simulink model "r5"  (Simulink 8.6)
settings: Solver=FixedStepAuto  StartTime=0.0  StopTime=10.0  RelTol=1e-3
undefined symbols (not defined in the file): dt, sldvsubsys, transition_v, transition_y
libraries: simulink x2, sldvlib x2
settings Model: Creator=elliocm  LastModifiedBy=mike
settings DebuggingCC: FcnCallInpInsideContextMsg=UseLocalSettings

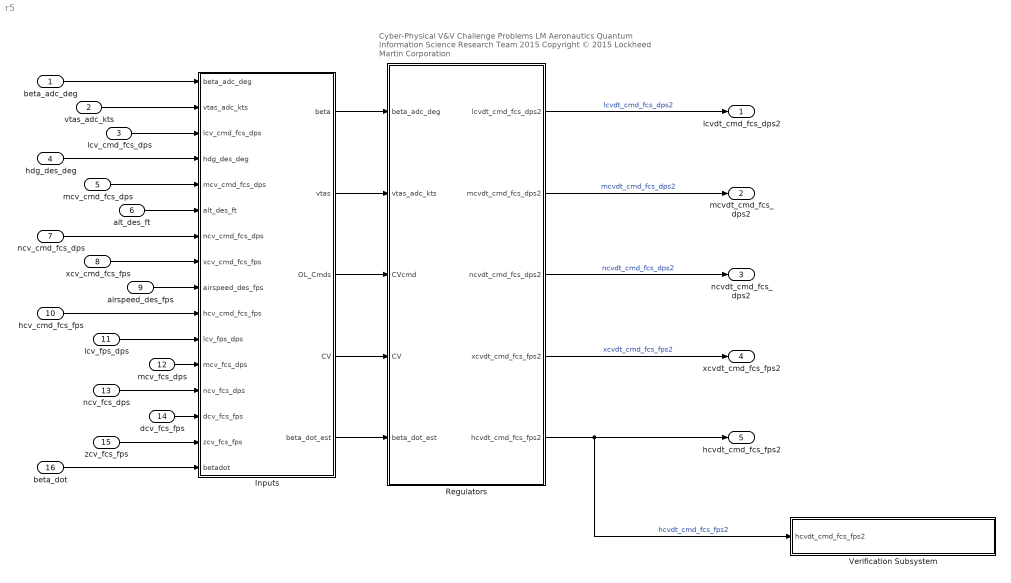
== system r5 ==
  note: Cyber-Physical V&V Challenge Problems
      | LM Aeronautics Quantum Information Science Research Team 2015
      | Copyright © 2015 Lockheed Martin Corporation
  beta_adc_deg : Inport  OutDataTypeStr=double
  vtas_adc_kts : Inport  Port=2  OutDataTypeStr=double
  "lcv_cmd_fcs_dps " : Inport  Port=3  OutDataTypeStr=double
  hdg_des_deg : Inport  Port=4  OutDataTypeStr=double
  mcv_cmd_fcs_dps : Inport  Port=5  OutDataTypeStr=double
  alt_des_ft : Inport  Port=6  OutDataTypeStr=double
  ncv_cmd_fcs_dps : Inport  Port=7  OutDataTypeStr=double
  xcv_cmd_fcs_fps : Inport  Port=8  OutDataTypeStr=double
  airspeed_des_fps : Inport  Port=9  OutDataTypeStr=double
  hcv_cmd_fcs_fps : Inport  Port=10  OutDataTypeStr=double
  lcv_fps_dps : Inport  Port=11  OutDataTypeStr=double
  mcv_fcs_dps : Inport  Port=12  OutDataTypeStr=double
  ncv_fcs_dps : Inport  Port=13  OutDataTypeStr=double
  dcv_fcs_fps : Inport  Port=14  OutDataTypeStr=double
  zcv_fcs_fps : Inport  Port=15  OutDataTypeStr=double
  beta_dot : Inport  Port=16  OutDataTypeStr=double
  Inputs : Subsystem
  Regulators : Subsystem
  Verification Subsystem : Subsystem  Tag=VerificationSubsystem  DisableCoverage=on  LoadFcn=sldvsubsys('check')  TreatAsAtomicUnit=on  SimViewingDevice=on  mask(VerificationSubsystem){}
      mask init:
      | sldvsubsys('maskInit');
      settings: CopyFcn=sldvsubsys('copy');  OpenFcn=open_system(gcb,'force');
      settings: PreSaveFcn=|
      | set_param(gcb,'SimViewingDevice','on');
      | sldvsubsys('check');
      mask Help: helpview(fullfile(docroot,'toolbox','sldv','sldv.map'),'verificationsubsystem')
      mask Display: image(imread('sldvicon_versubsys.png','BackGroundColor',[1 1 1]),'center');
  lcvdt_cmd_fcs_dps2 : Outport
  mcvdt_cmd_fcs_dps2 : Outport  Port=2
  ncvdt_cmd_fcs_dps2 : Outport  Port=3
  xcvdt_cmd_fcs_fps2 : Outport  Port=4
  hcvdt_cmd_fcs_fps2 : Outport  Port=5
  wires:
  Inputs/4(CV) -> Regulators/4(CV)
  Inputs/3(OL_Cmds) -> Regulators/3(CVcmd)
  Inputs/1(beta) -> Regulators/1(beta_adc_deg)
  Inputs/5(beta_dot_est) -> Regulators/5(beta_dot_est)
  beta_adc_deg/1 -> Inputs/1(beta_adc_deg)
  vtas_adc_kts/1 -> Inputs/2(vtas_adc_kts)
  "lcv_cmd_fcs_dps "/1 -> Inputs/3("lcv_cmd_fcs_dps ")
  mcv_cmd_fcs_dps/1 -> Inputs/5(mcv_cmd_fcs_dps)
  ncv_cmd_fcs_dps/1 -> Inputs/7(ncv_cmd_fcs_dps)
  xcv_cmd_fcs_fps/1 -> Inputs/8(xcv_cmd_fcs_fps)
  hcv_cmd_fcs_fps/1 -> Inputs/10(hcv_cmd_fcs_fps)
  hdg_des_deg/1 -> Inputs/4(hdg_des_deg)
  alt_des_ft/1 -> Inputs/6(alt_des_ft)
  airspeed_des_fps/1 -> Inputs/9(airspeed_des_fps)
  Regulators/1(lcvdt_cmd_fcs_dps2) -> lcvdt_cmd_fcs_dps2/1  "lcvdt_cmd_fcs_dps2"
  Regulators/2(mcvdt_cmd_fcs_dps2) -> mcvdt_cmd_fcs_dps2/1  "mcvdt_cmd_fcs_dps2"
  Regulators/3(ncvdt_cmd_fcs_dps2) -> ncvdt_cmd_fcs_dps2/1  "ncvdt_cmd_fcs_dps2"
  Regulators/5(hcvdt_cmd_fcs_fps2) -> Verification Subsystem/1(hcvdt_cmd_fcs_fps2), hcvdt_cmd_fcs_fps2/1  "hcvdt_cmd_fcs_fps2"
  Regulators/4(xcvdt_cmd_fcs_fps2) -> xcvdt_cmd_fcs_fps2/1  "xcvdt_cmd_fcs_fps2"
  zcv_fcs_fps/1 -> Inputs/15(zcv_fcs_fps)
  dcv_fcs_fps/1 -> Inputs/14(dcv_fcs_fps)
  lcv_fps_dps/1 -> Inputs/11(lcv_fps_dps)
  mcv_fcs_dps/1 -> Inputs/12(mcv_fcs_dps)
  ncv_fcs_dps/1 -> Inputs/13(ncv_fcs_dps)
  beta_dot/1 -> Inputs/16(betadot)
  Inputs/2(vtas) -> Regulators/2(vtas_adc_kts)

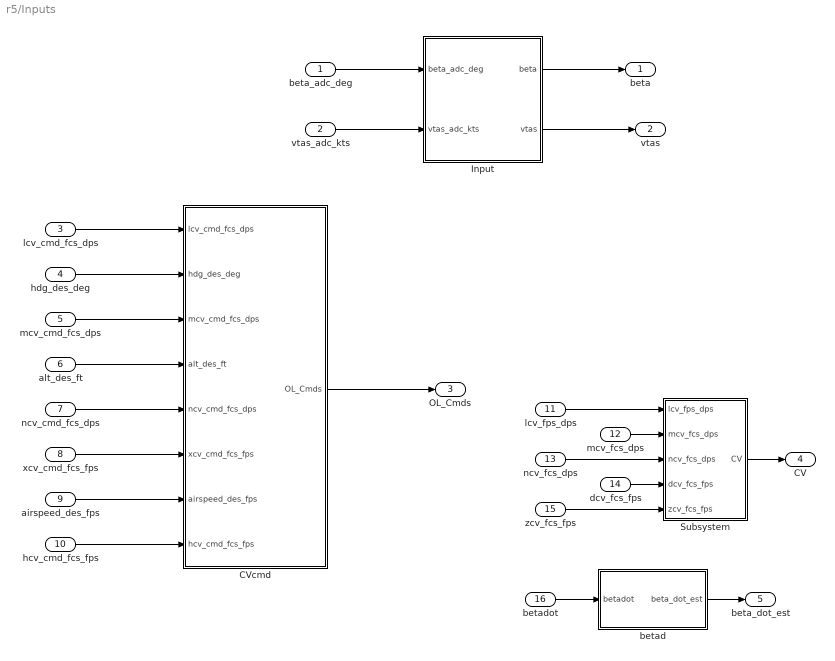
== system r5/Inputs ==
  beta_adc_deg : Inport
  vtas_adc_kts : Inport  Port=2
  "lcv_cmd_fcs_dps " : Inport  Port=3
  hdg_des_deg : Inport  Port=4
  mcv_cmd_fcs_dps : Inport  Port=5
  alt_des_ft : Inport  Port=6
  ncv_cmd_fcs_dps : Inport  Port=7
  xcv_cmd_fcs_fps : Inport  Port=8
  airspeed_des_fps : Inport  Port=9
  hcv_cmd_fcs_fps : Inport  Port=10
  lcv_fps_dps : Inport  Port=11
  mcv_fcs_dps : Inport  Port=12
  ncv_fcs_dps : Inport  Port=13
  dcv_fcs_fps : Inport  Port=14
  zcv_fcs_fps : Inport  Port=15
  betadot : Inport  Port=16
  CVcmd : Subsystem
  Input : Subsystem
  Subsystem : Subsystem
  betad : Subsystem
  beta : Outport
  vtas : Outport  Port=2
  OL_Cmds : Outport  Port=3
  CV : Outport  Port=4
  beta_dot_est : Outport  Port=5
  wires:
  Subsystem/1(CV) -> CV/1
  CVcmd/1(OL_Cmds) -> OL_Cmds/1
  beta_adc_deg/1 -> Input/1(beta_adc_deg)
  vtas_adc_kts/1 -> Input/2(vtas_adc_kts)
  "lcv_cmd_fcs_dps "/1 -> CVcmd/1("lcv_cmd_fcs_dps ")
  mcv_cmd_fcs_dps/1 -> CVcmd/3(mcv_cmd_fcs_dps)
  ncv_cmd_fcs_dps/1 -> CVcmd/5(ncv_cmd_fcs_dps)
  xcv_cmd_fcs_fps/1 -> CVcmd/6(xcv_cmd_fcs_fps)
  hcv_cmd_fcs_fps/1 -> CVcmd/8(hcv_cmd_fcs_fps)
  hdg_des_deg/1 -> CVcmd/2(hdg_des_deg)
  alt_des_ft/1 -> CVcmd/4(alt_des_ft)
  airspeed_des_fps/1 -> CVcmd/7(airspeed_des_fps)
  zcv_fcs_fps/1 -> Subsystem/5(zcv_fcs_fps)
  dcv_fcs_fps/1 -> Subsystem/4(dcv_fcs_fps)
  lcv_fps_dps/1 -> Subsystem/1(lcv_fps_dps)
  mcv_fcs_dps/1 -> Subsystem/2(mcv_fcs_dps)
  ncv_fcs_dps/1 -> Subsystem/3(ncv_fcs_dps)
  betadot/1 -> betad/1(betadot)
  betad/1(beta_dot_est) -> beta_dot_est/1
  Input/1(beta) -> beta/1
  Input/2(vtas) -> vtas/1

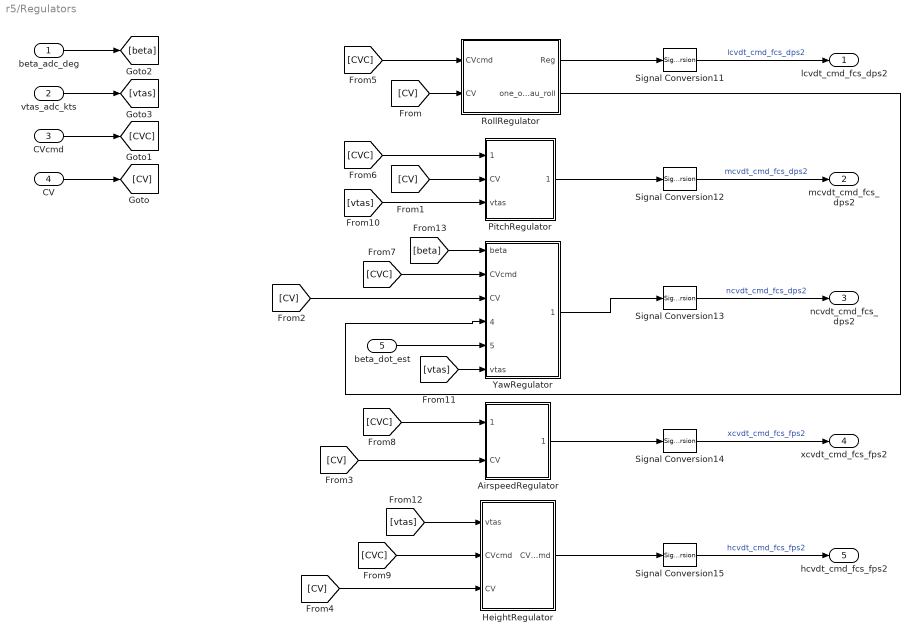
== system r5/Regulators ==
  beta_adc_deg : Inport
  vtas_adc_kts : Inport  Port=2
  CVcmd : Inport  Port=3
  CV : Inport  Port=4
  beta_dot_est : Inport  Port=5
  AirspeedRegulator : Subsystem
  HeightRegulator : Subsystem
  PitchRegulator : Subsystem
  RollRegulator : Subsystem
  Signal Conversion{11..15} (5 alike) : SignalConversion  ConversionOutput=Contiguous copy  OverrideOpt=on
  YawRegulator : Subsystem
  lcvdt_cmd_fcs_dps2 : Outport
  mcvdt_cmd_fcs_dps2 : Outport  Port=2
  ncvdt_cmd_fcs_dps2 : Outport  Port=3
  xcvdt_cmd_fcs_fps2 : Outport  Port=4
  hcvdt_cmd_fcs_fps2 : Outport  Port=5
  wires:
  RollRegulator/1(Reg) -> Signal Conversion11/1
  PitchRegulator/1(CVdt_cmd) -> Signal Conversion12/1
  YawRegulator/1(CVdt_cmd) -> Signal Conversion13/1
  AirspeedRegulator/1(CVdt_cmd) -> Signal Conversion14/1
  HeightRegulator/1(CVdt_cmd) -> Signal Conversion15/1
  [CVC] -> HeightRegulator/2(CVcmd)
  [CVC] -> YawRegulator/2(CVcmd)
  Signal Conversion11/1 -> lcvdt_cmd_fcs_dps2/1  "lcvdt_cmd_fcs_dps2"
  Signal Conversion12/1 -> mcvdt_cmd_fcs_dps2/1  "mcvdt_cmd_fcs_dps2"
  Signal Conversion13/1 -> ncvdt_cmd_fcs_dps2/1  "ncvdt_cmd_fcs_dps2"
  Signal Conversion15/1 -> hcvdt_cmd_fcs_fps2/1  "hcvdt_cmd_fcs_fps2"
  Signal Conversion14/1 -> xcvdt_cmd_fcs_fps2/1  "xcvdt_cmd_fcs_fps2"
  RollRegulator/2(one_over_Tau_roll) -> YawRegulator/4(one_over_Tau_roll)
  beta_dot_est/1 -> YawRegulator/5(beta_dot_est)
  CV/1 -> [CV]
  [CV] -> RollRegulator/2(CV)
  [CV] -> PitchRegulator/2(CV)
  [CV] -> YawRegulator/3(CV)
  [CV] -> AirspeedRegulator/2(CV)
  [CV] -> HeightRegulator/3(CV)
  CVcmd/1 -> [CVC]
  [CVC] -> RollRegulator/1(CVcmd)
  [CVC] -> PitchRegulator/1(CV_cmd)
  [CVC] -> AirspeedRegulator/1(CVcmd)
  [vtas] -> PitchRegulator/3(vtas)
  [vtas] -> HeightRegulator/1(vtas)
  beta_adc_deg/1 -> [beta]
  vtas_adc_kts/1 -> [vtas]
  [vtas] -> YawRegulator/6(vtas)
  [beta] -> YawRegulator/1(beta)

== system r5/Verification Subsystem ==
  note: The Inner Loop Height Regulator Shall not command translational height accelerations greater
      | than the capability of the system (32 ft/sec2) for durations exceeding 100 frames (1 second @ 100 hz).
  note: hcvdt_cmd_fcs_fps2{t}<=32 or hcvdt_cmd_fcs_fps2{t-1}<=32 or hcvdt_cmd_fcs_fps2{t-2}<=32 or hcvdt_cmd_fcs_fps2{t-3}<=32 or hcvdt_cmd_fcs_fps2{t-4}<=32 or hcvdt_cmd_fcs_fps2{t-5}<=32 or hcvdt_cmd_fcs_fps2{t-6}<=32 or hcvdt_cmd_fcs_fps2{t-7}<=32 or hcvdt_cmd_fcs_fps2{t-8}<=32 or hcvdt_cmd_fcs_fps2{t-9}<=32 or hcvdt_cmd_fcs_fps2{t-10}<=32 or hcvdt_cmd_fcs_fps2{t-11}<=32 or hcvdt_cmd_fcs_fps2{t-12}<=32 or hcvdt_cmd_fcs_fps2{t-13}<=32 or hcvdt_cmd_fcs_fps2{t-14}<=32 or hcvdt_cmd_fcs_fps2{t-15}<=32 or hcvdt_cmd_fcs_fps2{t-16}<=32 or hcvdt_cmd_fcs_fps2{t-17}<=32 or hcvdt_cmd_fcs_fps2{t-18}<=32 or hcvdt_cmd_fcs_fps2{t-19}<=32 or hcvdt_cmd_fcs_fps2{t-20}<=32 or hcvdt_cmd_fcs_fps2{t-21}<=32 or hcvdt_cmd_fcs_fps2{t-22}<=32 or hcvdt_cmd_fcs_fps2{t-23}<=32 or hcvdt_cmd_fcs_fps2{t-24}<=32 or hcvdt_cmd_fcs_fps2{t-25}<=32 or hcvdt_cmd_fcs_fps2{t-26}<=32 or hcvdt_cmd_fcs_fps2{t-27}<=32 or hcvdt_cmd_fcs_fps2{t-28}<=32 or hcvdt_cmd_fcs_fps2{t-29}<=32 or hcvdt_cmd_fcs_fps2{t-30}<=32 or hcvdt_cmd_fcs_fps2{t-31}<=32 or hcvdt_cmd_fcs_fps2{t-32}<=32 or hcvdt_cmd_fcs_fps2{t-33}<=32 or hcvdt_cmd_fcs_fps2{t-34}<=32 or hcvdt_cmd_fcs_fps2{t-35}<=32 or hcvdt_cmd_fcs_fps2{t-36}<=32 or hcvdt_cmd_fcs_fps2{t-37}<=32 or hcvdt_cmd_fcs_fps2{t-38}<=32 or hcvdt_cmd_fcs_fps2{t-39}<=32 or hcvdt_cmd_fcs_fps2{t-40}<=32 or hcvdt_cmd_fcs_fps2{t-41}<=32 or hcvdt_cmd_fcs_fps2{t-42}<=32 or hcvdt_cmd_fcs_fps2{t-43}<=32 or hcvdt_cmd_fcs_fps2{t-44}<=32 or hcvdt_cmd_fcs_fps2{t-45}<=32 or hcvdt_cmd_fcs_fps2{t-46}<=32 or hcvdt_cmd_fcs_fps2{t-47}<=32 or hcvdt_cmd_fcs_fps2{t-48}<=32 or hcvdt_cmd_fcs_fps2{t-49}<=32 or hcvdt_cmd_fcs_fps2{t-32}<=32 or hcvdt_cmd_fcs_fps2{t-51}<=32 or hcvdt_cmd_fcs_fps2{t-52}<=32 or hcvdt_cmd_fcs_fps2{t-53}<=32 or hcvdt_cmd_fcs_fps2{t-54}<=32 or hcvdt_cmd_fcs_fps2{t-55}<=32 or hcvdt_cmd_fcs_fps2{t-56}<=32 or hcvdt_cmd_fcs_fps2{t-57}<=32 or hcvdt_cmd_fcs_fps2{t-58}<=32 or hcvdt_cmd_fcs_fps2{t-59}<=32 or hcvdt_cmd_fcs_fps2{t-60}<=32 or hcvdt_cmd_fcs_fps2{t-61}<=32 or hcvdt_cmd_fcs_fps2{t-62}<=32 or hcvdt_cmd_fcs_fps2{t-63}<=32 or hcvdt_cmd_fcs_fps2{t-64}<=32 or hcvdt_cmd_fcs_fps2{t-65}<=32 or hcvdt_cmd_fcs_fps2{t-66}<=32 or hcvdt_cmd_fcs_fps2{t-67}<=32 or hcvdt_cmd_fcs_fps2{t-68}<=32 or hcvdt_cmd_fcs_fps2{t-69}<=32 or hcvdt_cmd_fcs_fps2{t-70}<=32 or hcvdt_cmd_fcs_fps2{t-71}<=32 or hcvdt_cmd_fcs_fps2{t-72}<=32 or hcvdt_cmd_fcs_fps2{t-73}<=32 or hcvdt_cmd_fcs_fps2{t-74}<=32 or hcvdt_cmd_fcs_fps2{t-75}<=32 or hcvdt_cmd_fcs_fps2{t-76}<=32 or hcvdt_cmd_fcs_fps2{t-77}<=32 or hcvdt_cmd_fcs_fps2{t-78}<=32 or hcvdt_cmd_fcs_fps2{t-79}<=32 or hcvdt_cmd_fcs_fps2{t-80}<=32 or hcvdt_cmd_fcs_fps2{t-81}<=32 or hcvdt_cmd_fcs_fps2{t-82}<=32 or hcvdt_cmd_fcs_fps2{t-83}<=32 or hcvdt_cmd_fcs_fps2{t-84}<=32 or hcvdt_cmd_fcs_fps2{t-85}<=32 or hcvdt_cmd_fcs_fps2{t-86}<=32 or hcvdt_cmd_fcs_fps2{t-87}<=32 or hcvdt_cmd_fcs_fps2{t-88}<=32 or hcvdt_cmd_fcs_fps2{t-89}<=32 or hcvdt_cmd_fcs_fps2{t-90}<=32 or hcvdt_cmd_fcs_fps2{t-91}<=32 or hcvdt_cmd_fcs_fps2{t-92}<=32 or hcvdt_cmd_fcs_fps2{t-93}<=32 or hcvdt_cmd_fcs_fps2{t-94}<=32 or hcvdt_cmd_fcs_fps2{t-95}<=32 or hcvdt_cmd_fcs_fps2{t-96}<=32 or hcvdt_cmd_fcs_fps2{t-97}<=32 or hcvdt_cmd_fcs_fps2{t-98}<=32 or hcvdt_cmd_fcs_fps2{t-99}<=32;
  hcvdt_cmd_fcs_fps2 : Inport
  Constant : Constant  Value=32
  Detector : sldvlib/Temporal Operators/Detector  reset=off  typ=Synchronized  in_hold=100  delay=1  out_hold=3
  Logical Operator : Logic  Operator=NOT  AllPortsSameDT=off  OutDataTypeStr=boolean
  Proof Objective : sldvlib/Objectives and Constraints/Proof Objective  enabled=on  customAVTBlockType=Proof Objective  intervals=true  dispValues=on  outEnabled=off  enableStopSim=off
      settings: AttributesFormatString=%<intervals>
  Relational Operator : RelationalOperator  Operator=>  OutDataTypeStr=boolean
  wires:
  Relational Operator/1 -> Detector/1
  hcvdt_cmd_fcs_fps2/1 -> Relational Operator/1
  Constant/1 -> Relational Operator/2
  Logical Operator/1 -> Proof Objective/1
  Detector/1 -> Logical Operator/1

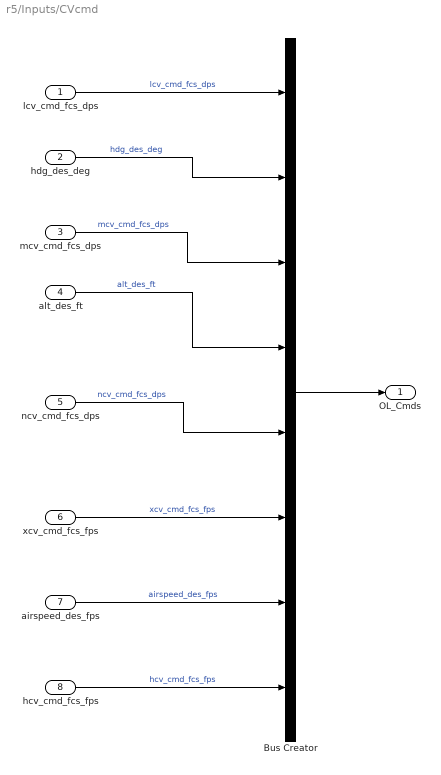
== system r5/Inputs/CVcmd ==
  "lcv_cmd_fcs_dps " : Inport
  hdg_des_deg : Inport  Port=2
  mcv_cmd_fcs_dps : Inport  Port=3
  alt_des_ft : Inport  Port=4
  ncv_cmd_fcs_dps : Inport  Port=5
  xcv_cmd_fcs_fps : Inport  Port=6
  airspeed_des_fps : Inport  Port=7
  hcv_cmd_fcs_fps : Inport  Port=8
  Bus Creator : BusCreator  Inputs=8
  OL_Cmds : Outport
  wires:
  "lcv_cmd_fcs_dps "/1 -> Bus Creator/1  "lcv_cmd_fcs_dps"
  mcv_cmd_fcs_dps/1 -> Bus Creator/3  "mcv_cmd_fcs_dps"
  ncv_cmd_fcs_dps/1 -> Bus Creator/5  "ncv_cmd_fcs_dps"
  xcv_cmd_fcs_fps/1 -> Bus Creator/6  "xcv_cmd_fcs_fps"
  hcv_cmd_fcs_fps/1 -> Bus Creator/8  "hcv_cmd_fcs_fps"
  Bus Creator/1 -> OL_Cmds/1
  hdg_des_deg/1 -> Bus Creator/2  "hdg_des_deg"
  alt_des_ft/1 -> Bus Creator/4  "alt_des_ft"
  airspeed_des_fps/1 -> Bus Creator/7  "airspeed_des_fps"

== system r5/Inputs/Input ==
  beta_adc_deg : Inport
  vtas_adc_kts : Inport  Port=2
  egi_fcs_in : Subsystem
  beta : Outport
  vtas : Outport  Port=2
  wires:
  beta_adc_deg/1 -> egi_fcs_in/1(beta_adc_deg)  "beta_adc_deg"
  vtas_adc_kts/1 -> egi_fcs_in/2(vtas_adc_kts)  "vtas_adc_kts"
  egi_fcs_in/1(beta_deg) -> beta/1
  egi_fcs_in/2(vtas_kts) -> vtas/1

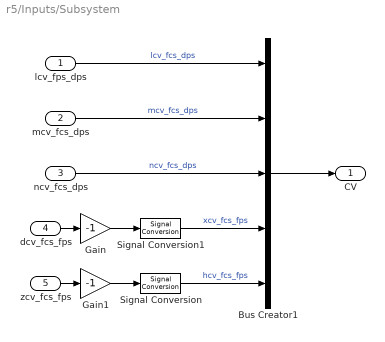
== system r5/Inputs/Subsystem ==
  lcv_fps_dps : Inport
  mcv_fcs_dps : Inport  Port=2
  ncv_fcs_dps : Inport  Port=3
  dcv_fcs_fps : Inport  Port=4
  zcv_fcs_fps : Inport  Port=5
  Bus Creator1 : BusCreator  Inputs=5
  Gain : Gain  Gain=-1
  Gain1 : Gain  Gain=-1
  Signal Conversion : SignalConversion  ConversionOutput=Contiguous copy
  Signal Conversion1 : SignalConversion  ConversionOutput=Contiguous copy
  CV : Outport
  wires:
  Gain1/1 -> Signal Conversion/1
  zcv_fcs_fps/1 -> Gain1/1
  Signal Conversion1/1 -> Bus Creator1/4  "xcv_fcs_fps"
  Gain/1 -> Signal Conversion1/1
  Bus Creator1/1 -> CV/1
  mcv_fcs_dps/1 -> Bus Creator1/2  "mcv_fcs_dps"
  lcv_fps_dps/1 -> Bus Creator1/1  "lcv_fcs_dps"
  Signal Conversion/1 -> Bus Creator1/5  "hcv_fcs_fps"
  ncv_fcs_dps/1 -> Bus Creator1/3  "ncv_fcs_dps"
  dcv_fcs_fps/1 -> Gain/1

== system r5/Inputs/betad ==
  betadot : Inport
  beta_dot_est : Outport
  wires:
  betadot/1 -> beta_dot_est/1

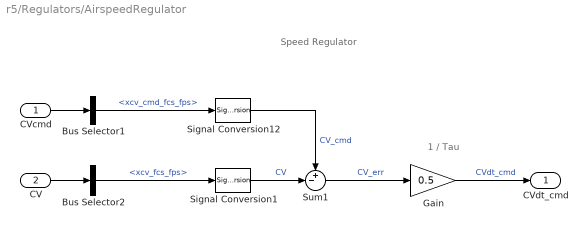
== system r5/Regulators/AirspeedRegulator ==
  note: Speed Regulator
  note: 1 / Tau
  CVcmd : Inport
  CV : Inport  Port=2
  Bus Selector1 : BusSelector  OutputSignals=xcv_cmd_fcs_fps
  Bus Selector2 : BusSelector  OutputSignals=xcv_fcs_fps
  Gain : Gain  Gain=0.5
  Signal Conversion1 : SignalConversion  ConversionOutput=Contiguous copy  OverrideOpt=on
  Signal Conversion12 : SignalConversion  ConversionOutput=Contiguous copy  OverrideOpt=on
  Sum1 : Sum  Inputs=+-|  SaturateOnIntegerOverflow=on  InputSameDT=on  OutDataTypeStr=Inherit: Same as first input
  CVdt_cmd : Outport
  wires:
  Gain/1 -> CVdt_cmd/1  "CVdt_cmd"
  CVcmd/1 -> Bus Selector1/1
  Signal Conversion12/1 -> Sum1/1  "CV_cmd"
  Signal Conversion1/1 -> Sum1/2  "CV"
  CV/1 -> Bus Selector2/1
  Bus Selector2/1 -> Signal Conversion1/1  "<xcv_fcs_fps>"
  Bus Selector1/1 -> Signal Conversion12/1  "<xcv_cmd_fcs_fps>"
  Sum1/1 -> Gain/1  "CV_err"

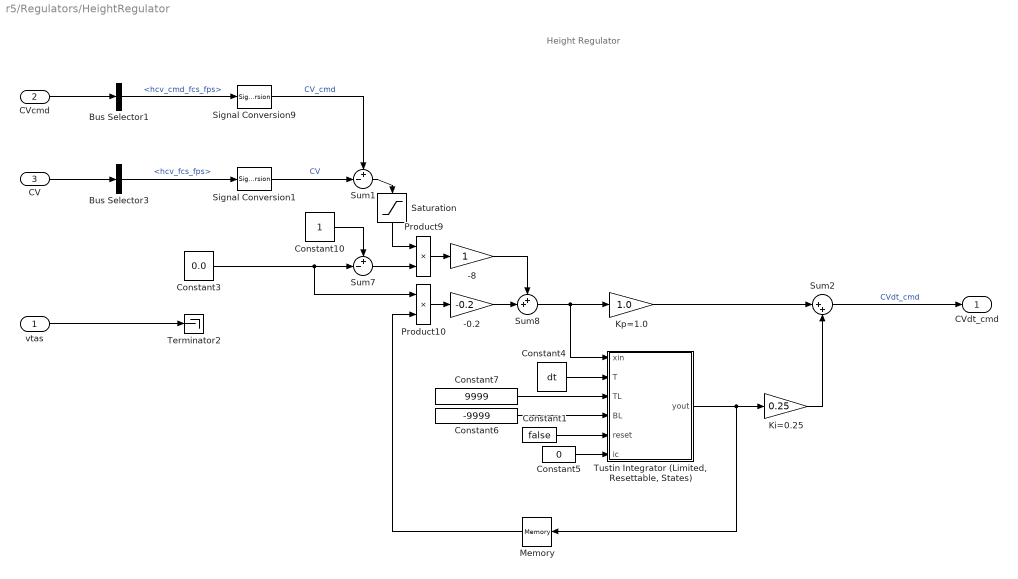
== system r5/Regulators/HeightRegulator ==
  note: Height Regulator
  vtas : Inport
  CVcmd : Inport  Port=2
  CV : Inport  Port=3
  -0.2 : Gain  Gain=-0.2
  -8 : Gain
  Bus Selector1 : BusSelector  OutputSignals=hcv_cmd_fcs_fps
  Bus Selector3 : BusSelector  OutputSignals=hcv_fcs_fps
  Constant1 : Constant  Value=false
  Constant10 : Constant
  Constant3 : Constant  Value=0.0
  Constant4 : Constant  Value=dt
  Constant5 : Constant  Value=0
  Constant6 : Constant  Value=-9999
  Constant7 : Constant  Value=9999
  Ki=0.25 : Gain  Gain=0.25
  Kp=1.0 : Gain  Gain=1.0
  Memory : Memory
  Product10 : Product  SaturateOnIntegerOverflow=on  OutDataTypeStr=Inherit: Same as first input
  Product9 : Product  SaturateOnIntegerOverflow=on  OutDataTypeStr=Inherit: Same as first input
  Saturation : Saturate  UpperLimit=1  LowerLimit=-1
  Signal Conversion1 : SignalConversion  ConversionOutput=Contiguous copy  OverrideOpt=on
  Signal Conversion9 : SignalConversion  ConversionOutput=Contiguous copy  OverrideOpt=on
  Sum1 : Sum  Inputs=+-|  SaturateOnIntegerOverflow=on  InputSameDT=on  OutDataTypeStr=Inherit: Same as first input
  Sum2 : Sum  Inputs=|++  SaturateOnIntegerOverflow=on  InputSameDT=on  OutDataTypeStr=Inherit: Same as first input
  Sum7 : Sum  Inputs=+-|
  Sum8 : Sum  Inputs=++|
  Terminator2 : Terminator
  "Tustin Integrator (Limited, Resettable, States)" : Subsystem
  CVdt_cmd : Outport
  wires:
  Bus Selector1/1 -> Signal Conversion9/1  "<hcv_cmd_fcs_fps>"
  CVcmd/1 -> Bus Selector1/1
  Signal Conversion9/1 -> Sum1/1  "CV_cmd"
  Signal Conversion1/1 -> Sum1/2  "CV"
  CV/1 -> Bus Selector3/1
  Bus Selector3/1 -> Signal Conversion1/1  "<hcv_fcs_fps>"
  Sum1/1 -> Saturation/1
  Sum2/1 -> CVdt_cmd/1  "CVdt_cmd"
  Ki=0.25/1 -> Sum2/2
  Kp=1.0/1 -> Sum2/1
  Product9/1 -> -8/1
  Product10/1 -> -0.2/1
  -0.2/1 -> Sum8/2
  -8/1 -> Sum8/1
  Sum7/1 -> Product9/2
  Constant3/1 -> Sum7/2, Product10/1
  Constant10/1 -> Sum7/1
  Sum8/1 -> "Tustin Integrator (Limited, Resettable, States)"/1(xin), Kp=1.0/1
  Memory/1 -> Product10/2
  vtas/1 -> Terminator2/1
  Saturation/1 -> Product9/1
  Constant4/1 -> "Tustin Integrator (Limited, Resettable, States)"/2(T)
  Constant7/1 -> "Tustin Integrator (Limited, Resettable, States)"/3(TL)
  Constant6/1 -> "Tustin Integrator (Limited, Resettable, States)"/4(BL)
  Constant1/1 -> "Tustin Integrator (Limited, Resettable, States)"/5(reset)
  Constant5/1 -> "Tustin Integrator (Limited, Resettable, States)"/6(ic)
  "Tustin Integrator (Limited, Resettable, States)"/1(yout) -> Memory/1, Ki=0.25/1

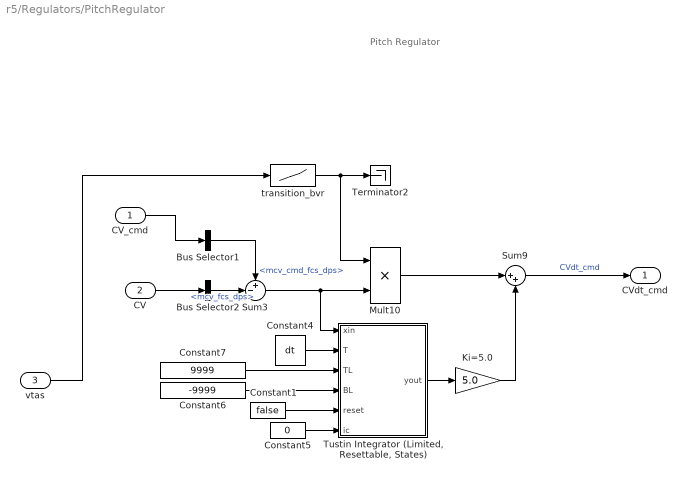
== system r5/Regulators/PitchRegulator ==
  note: Pitch Regulator
  CV_cmd : Inport
  CV : Inport  Port=2
  vtas : Inport  Port=3
  Bus Selector1 : BusSelector  OutputSignals=mcv_cmd_fcs_dps
  Bus Selector2 : BusSelector  OutputSignals=mcv_fcs_dps
  Constant1 : Constant  Value=false
  Constant4 : Constant  Value=dt
  Constant5 : Constant  Value=0
  Constant6 : Constant  Value=-9999
  Constant7 : Constant  Value=9999
  Ki=5.0 : Gain  Gain=5.0
  Mult10 : Product  SaturateOnIntegerOverflow=on  InputSameDT=on  OutDataTypeStr=Inherit: Same as first input
  Sum3 : Sum  Inputs=+-|  SaturateOnIntegerOverflow=on  InputSameDT=on  OutDataTypeStr=Inherit: Same as first input
  Sum9 : Sum  Inputs=|++  SaturateOnIntegerOverflow=on  InputSameDT=on  OutDataTypeStr=Inherit: Same as first input
  Terminator2 : Terminator
  "Tustin Integrator (Limited, Resettable, States)" : Subsystem
  transition_bvr : Lookup  InputValues=[120 185]  Table=[15 20]
  CVdt_cmd : Outport
  wires:
  CV_cmd/1 -> Bus Selector1/1
  CV/1 -> Bus Selector2/1
  Constant4/1 -> "Tustin Integrator (Limited, Resettable, States)"/2(T)
  Constant5/1 -> "Tustin Integrator (Limited, Resettable, States)"/6(ic)
  "Tustin Integrator (Limited, Resettable, States)"/1(yout) -> Ki=5.0/1
  Mult10/1 -> Sum9/1
  Ki=5.0/1 -> Sum9/2
  Sum9/1 -> CVdt_cmd/1  "CVdt_cmd"
  Bus Selector1/1 -> Sum3/1  "<mcv_cmd_fcs_dps>"
  Bus Selector2/1 -> Sum3/2  "<mcv_fcs_dps>"
  transition_bvr/1 -> Terminator2/1, Mult10/1
  Constant1/1 -> "Tustin Integrator (Limited, Resettable, States)"/5(reset)
  vtas/1 -> transition_bvr/1
  Sum3/1 -> "Tustin Integrator (Limited, Resettable, States)"/1(xin), Mult10/2
  Constant6/1 -> "Tustin Integrator (Limited, Resettable, States)"/4(BL)
  Constant7/1 -> "Tustin Integrator (Limited, Resettable, States)"/3(TL)

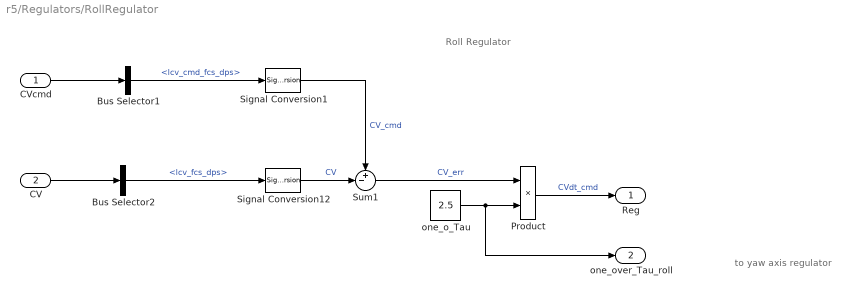
== system r5/Regulators/RollRegulator ==
  note: Roll Regulator
  note: to yaw axis regulator
  CVcmd : Inport
  CV : Inport  Port=2
  Bus Selector1 : BusSelector  OutputSignals=lcv_cmd_fcs_dps
  Bus Selector2 : BusSelector  OutputSignals=lcv_fcs_dps
  Product : Product  RndMeth=Zero
  Signal Conversion1 : SignalConversion  ConversionOutput=Contiguous copy  OverrideOpt=on
  Signal Conversion12 : SignalConversion  ConversionOutput=Contiguous copy  OverrideOpt=on
  Sum1 : Sum  Inputs=+-|  SaturateOnIntegerOverflow=on  InputSameDT=on  OutDataTypeStr=Inherit: Same as first input
  one_o_Tau : Constant  Value=2.5
  Reg : Outport
  one_over_Tau_roll : Outport  Port=2
  wires:
  Sum1/1 -> Product/1  "CV_err"
  Signal Conversion1/1 -> Sum1/1  "CV_cmd"
  Signal Conversion12/1 -> Sum1/2  "CV"
  CV/1 -> Bus Selector2/1
  Bus Selector2/1 -> Signal Conversion12/1  "<lcv_fcs_dps>"
  Bus Selector1/1 -> Signal Conversion1/1  "<lcv_cmd_fcs_dps>"
  CVcmd/1 -> Bus Selector1/1
  one_o_Tau/1 -> Product/2, one_over_Tau_roll/1
  Product/1 -> Reg/1  "CVdt_cmd"

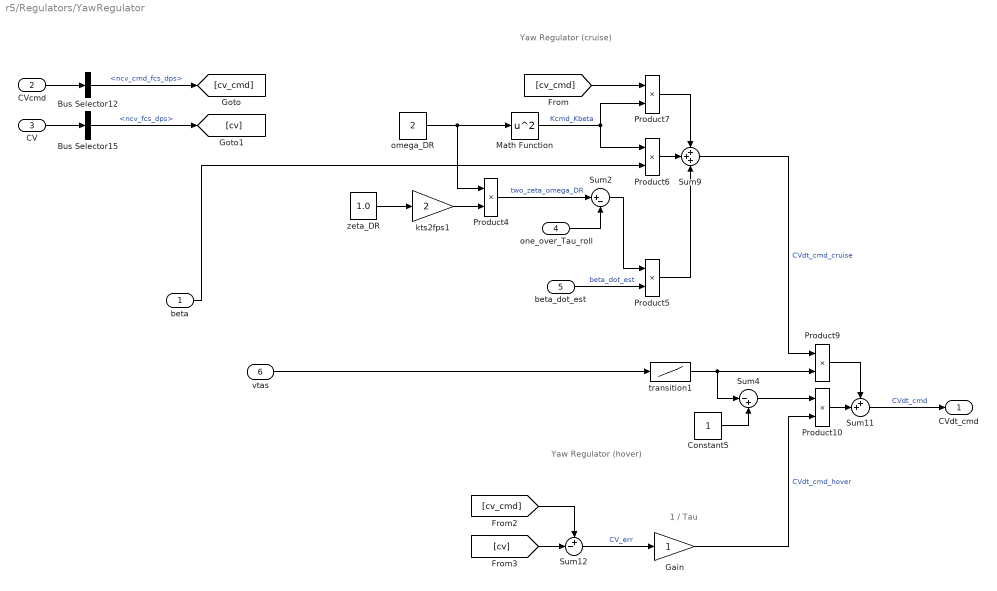
== system r5/Regulators/YawRegulator ==
  note: Yaw Regulator (hover)
  note: 1 / Tau
  note: Yaw Regulator (cruise)
  beta : Inport
  CVcmd : Inport  Port=2
  CV : Inport  Port=3
  one_over_Tau_roll : Inport  Port=4
  beta_dot_est : Inport  Port=5
  vtas : Inport  Port=6
  Bus Selector12 : BusSelector  OutputSignals=ncv_cmd_fcs_dps
  Bus Selector15 : BusSelector  OutputSignals=ncv_fcs_dps
  Constant5 : Constant
  Gain : Gain
  Math Function : Math  Operator=square  SaturateOnIntegerOverflow=on
  Product{4..7,9..10} (6 alike) : Product  SaturateOnIntegerOverflow=on  OutDataTypeStr=Inherit: Same as first input
  Sum11 : Sum  Inputs=++|
  Sum12 : Sum  Inputs=+-|  SaturateOnIntegerOverflow=on  InputSameDT=on  OutDataTypeStr=Inherit: Same as first input
  Sum2 : Sum  Inputs=|+-  SaturateOnIntegerOverflow=on  InputSameDT=on  OutDataTypeStr=Inherit: Same as first input
  Sum4 : Sum  Inputs=|-+
  Sum9 : Sum  Inputs=+++  SaturateOnIntegerOverflow=on  InputSameDT=on  OutDataTypeStr=Inherit: Same as first input
  kts2fps1 : Gain  Gain=2
  omega_DR : Constant  Value=2
  transition1 : Lookup  InputValues=transition_v  Table=transition_y
  zeta_DR : Constant  Value=1.0
  CVdt_cmd : Outport
  wires:
  beta/1 -> Product6/2
  Product6/1 -> Sum9/2
  omega_DR/1 -> Math Function/1, Product4/1
  Product7/1 -> Sum9/1
  Math Function/1 -> Product6/1, Product7/2  "Kcmd_Kbeta"
  Sum11/1 -> CVdt_cmd/1  "CVdt_cmd"
  transition1/1 -> Sum4/1, Product9/2
  Product9/1 -> Sum11/1
  Constant5/1 -> Sum4/2
  Sum4/1 -> Product10/1
  Product10/1 -> Sum11/2
  Sum9/1 -> Product9/1  "CVdt_cmd_cruise"
  Sum12/1 -> Gain/1  "CV_err"
  Bus Selector12/1 -> [cv_cmd]  "<ncv_cmd_fcs_dps>"
  CVcmd/1 -> Bus Selector12/1
  CV/1 -> Bus Selector15/1
  Bus Selector15/1 -> [cv]  "<ncv_fcs_dps>"
  beta_dot_est/1 -> Product5/2  "beta_dot_est"
  Gain/1 -> Product10/2  "CVdt_cmd_hover"
  [cv_cmd] -> Product7/1
  [cv_cmd] -> Sum12/1
  [cv] -> Sum12/2
  zeta_DR/1 -> kts2fps1/1
  kts2fps1/1 -> Product4/2
  Product4/1 -> Sum2/1  "two_zeta_omega_DR"
  one_over_Tau_roll/1 -> Sum2/2
  Product5/1 -> Sum9/3
  Sum2/1 -> Product5/1
  vtas/1 -> transition1/1

== system r5/Inputs/Input/egi_fcs_in ==
  beta_adc_deg : Inport
  vtas_adc_kts : Inport  Port=2
  beta_deg : Outport
  vtas_kts : Outport  Port=2
  wires:
  beta_adc_deg/1 -> beta_deg/1  "beta_adc_deg"
  vtas_adc_kts/1 -> vtas_kts/1  "vtas_adc_kts"

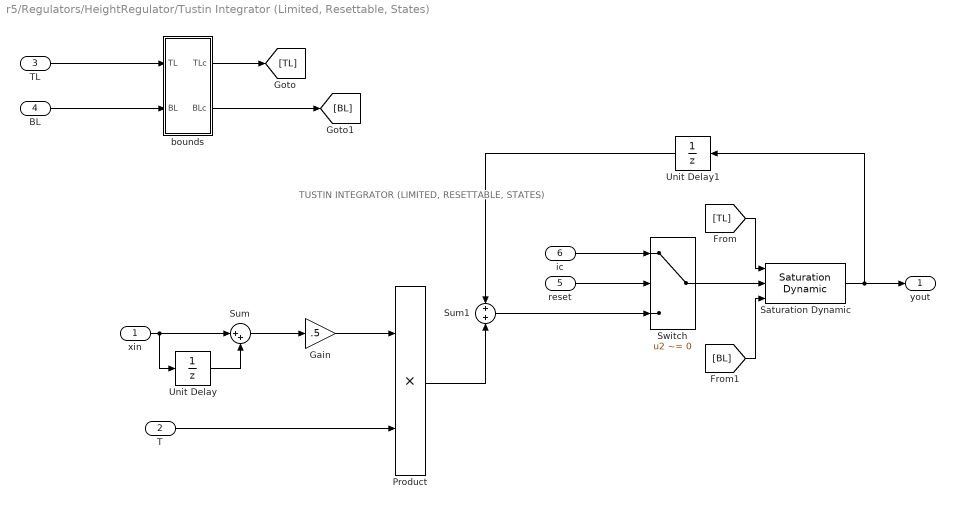
== system r5/Regulators/HeightRegulator/Tustin Integrator (Limited, Resettable, States) ==
  note: TUSTIN INTEGRATOR (LIMITED, RESETTABLE, STATES)
  xin : Inport
  T : Inport  Port=2
  TL : Inport  Port=3
  BL : Inport  Port=4
  reset : Inport  Port=5
  ic : Inport  Port=6
  Gain : Gain  Gain=.5
  Product : Product  RndMeth=Zero
  Saturation Dynamic : simulink/Discontinuities/Saturation Dynamic  OutMin=[]  OutMax=[]  OutDataTypeStr=Inherit: Same as second input  OutDataType=fixdt(1, 16)  OutScaling=2^-10  DoSatur=off
  Sum : Sum  Inputs=|++
  Sum1 : Sum
  Switch : Switch  Criteria=u2 ~= 0  Threshold=0.5
  Unit Delay : UnitDelay  SampleTime=-1
  Unit Delay1 : UnitDelay  SampleTime=-1
  bounds : Subsystem
  yout : Outport
  wires:
  xin/1 -> Unit Delay/1, Sum/1
  Unit Delay/1 -> Sum/2
  Sum/1 -> Gain/1
  Gain/1 -> Product/1
  T/1 -> Product/2
  Product/1 -> Sum1/2
  Sum1/1 -> Switch/3
  reset/1 -> Switch/2
  ic/1 -> Switch/1
  Switch/1 -> Saturation Dynamic/2
  Saturation Dynamic/1 -> Unit Delay1/1, yout/1
  Unit Delay1/1 -> Sum1/1
  TL/1 -> bounds/1(TL)
  BL/1 -> bounds/2(BL)
  bounds/1(TLc) -> [TL]
  bounds/2(BLc) -> [BL]
  [TL] -> Saturation Dynamic/1
  [BL] -> Saturation Dynamic/3

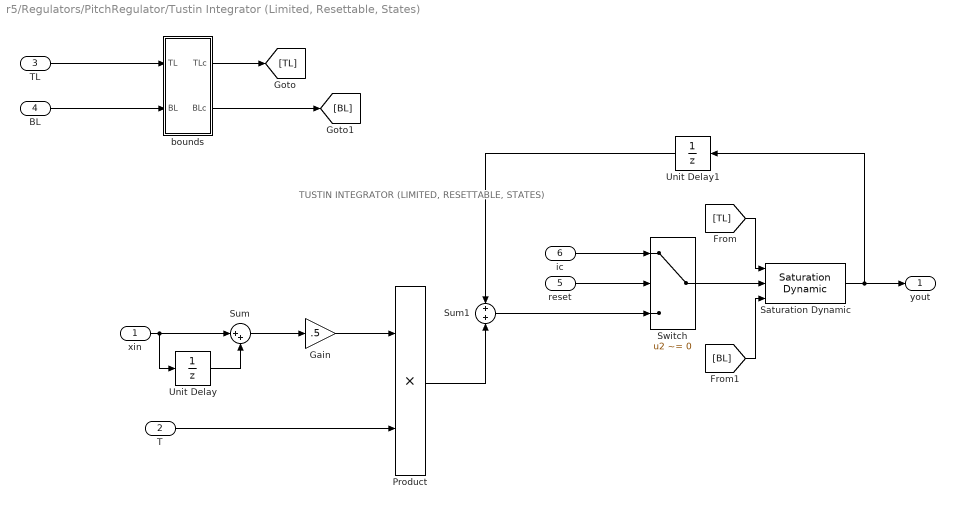
== system r5/Regulators/PitchRegulator/Tustin Integrator (Limited, Resettable, States) ==
  note: TUSTIN INTEGRATOR (LIMITED, RESETTABLE, STATES)
  xin : Inport
  T : Inport  Port=2
  TL : Inport  Port=3
  BL : Inport  Port=4
  reset : Inport  Port=5
  ic : Inport  Port=6
  Gain : Gain  Gain=.5
  Product : Product  RndMeth=Zero
  Saturation Dynamic : simulink/Discontinuities/Saturation Dynamic  OutMin=[]  OutMax=[]  OutDataTypeStr=Inherit: Same as second input  OutDataType=fixdt(1, 16)  OutScaling=2^-10  DoSatur=off
  Sum : Sum  Inputs=|++
  Sum1 : Sum
  Switch : Switch  Criteria=u2 ~= 0  Threshold=0.5
  Unit Delay : UnitDelay  SampleTime=-1
  Unit Delay1 : UnitDelay  SampleTime=-1
  bounds : Subsystem
  yout : Outport
  wires:
  xin/1 -> Unit Delay/1, Sum/1
  Unit Delay/1 -> Sum/2
  Sum/1 -> Gain/1
  Gain/1 -> Product/1
  T/1 -> Product/2
  Product/1 -> Sum1/2
  Sum1/1 -> Switch/3
  reset/1 -> Switch/2
  ic/1 -> Switch/1
  Switch/1 -> Saturation Dynamic/2
  Saturation Dynamic/1 -> Unit Delay1/1, yout/1
  Unit Delay1/1 -> Sum1/1
  TL/1 -> bounds/1(TL)
  BL/1 -> bounds/2(BL)
  bounds/1(TLc) -> [TL]
  bounds/2(BLc) -> [BL]
  [TL] -> Saturation Dynamic/1
  [BL] -> Saturation Dynamic/3

== system r5/Regulators/HeightRegulator/Tustin Integrator (Limited, Resettable, States)/bounds ==
  TL : Inport
  BL : Inport  Port=2
  Relational Operator : RelationalOperator  Operator=<  OutDataTypeStr=boolean
  Switch1 : Switch  Criteria=u2 ~= 0  Threshold=0.5
  Switch2 : Switch  Criteria=u2 ~= 0  Threshold=0.5
  TLc : Outport
  BLc : Outport  Port=2
  wires:
  BL/1 -> Switch1/1, Switch2/3, Relational Operator/2
  TL/1 -> Switch2/1, Switch1/3, Relational Operator/1
  Relational Operator/1 -> Switch2/2, Switch1/2
  Switch1/1 -> TLc/1
  Switch2/1 -> BLc/1

== system r5/Regulators/PitchRegulator/Tustin Integrator (Limited, Resettable, States)/bounds ==
  TL : Inport
  BL : Inport  Port=2
  Relational Operator : RelationalOperator  Operator=<  OutDataTypeStr=boolean
  Switch1 : Switch  Criteria=u2 ~= 0  Threshold=0.5
  Switch2 : Switch  Criteria=u2 ~= 0  Threshold=0.5
  TLc : Outport
  BLc : Outport  Port=2
  wires:
  BL/1 -> Switch1/1, Switch2/3, Relational Operator/2
  TL/1 -> Switch2/1, Switch1/3, Relational Operator/1
  Relational Operator/1 -> Switch2/2, Switch1/2
  Switch1/1 -> TLc/1
  Switch2/1 -> BLc/1
